simulink model "TubeFurnaceSim_2023b"  (R2023b)
settings: Solver=VariableStepAuto  StartTime=0.0  StopTime=240  FixedStep=0.001  RelTol=1e-3
values from neighbouring files (symbols this model uses):
  a_density = 1.225    [TubeFurnace.m]
  a_heat_cap = 1005    [TubeFurnace.m]
  ambient_temp = 25    [TubeFurnace.m]
  current = 15    [TubeFurnace.m]
  g = 9.81    [TubeFurnace.m]
  heat_eff = 0.85    [TubeFurnace.m]
  i_resist_cond = log((q_inner_dia/2 + i_thickness) / (q_inner_dia/2)) / (2*pi*i_therm_cond*q_length)    [TubeFurnace.m]
  k_d = 0    [TubeFurnace.m]
  k_i = 0    [TubeFurnace.m]
  k_p = 0.5    [TubeFurnace.m]
  q_emis = 0.8    [TubeFurnace.m]
  q_inner_dia = 20    [TubeFurnace.m]
  q_inner_sa = q_length * pi * (q_inner_dia / 2000)    (= 0.00957557440814)    [TubeFurnace.m]
  q_length = 1 * ft_to_m    (= 0.3048)    [TubeFurnace.m]
  stefan = 5.67*10^-8    (= 5.67e-08)    [TubeFurnace.m]
  w_tot_resist = w_resist * w_length / 100    (= 6.56167979003)    [TubeFurnace.m]
libraries: slpidlib x1
settings Model: Creator=Jason Kwok  LastModifiedBy=jason
settings RTWCC: GPUComputeCapability=5.0

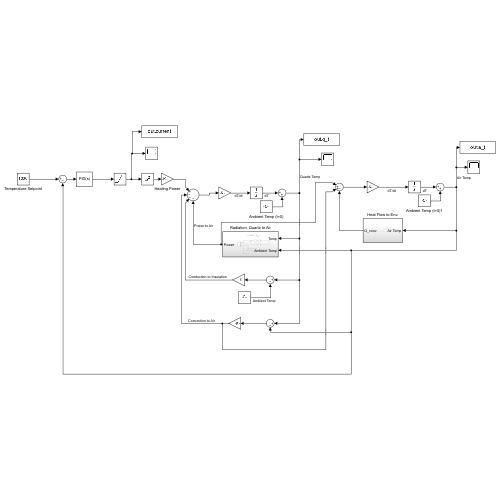
[thumbnail: Simulink's stored preview of the top-level diagram]
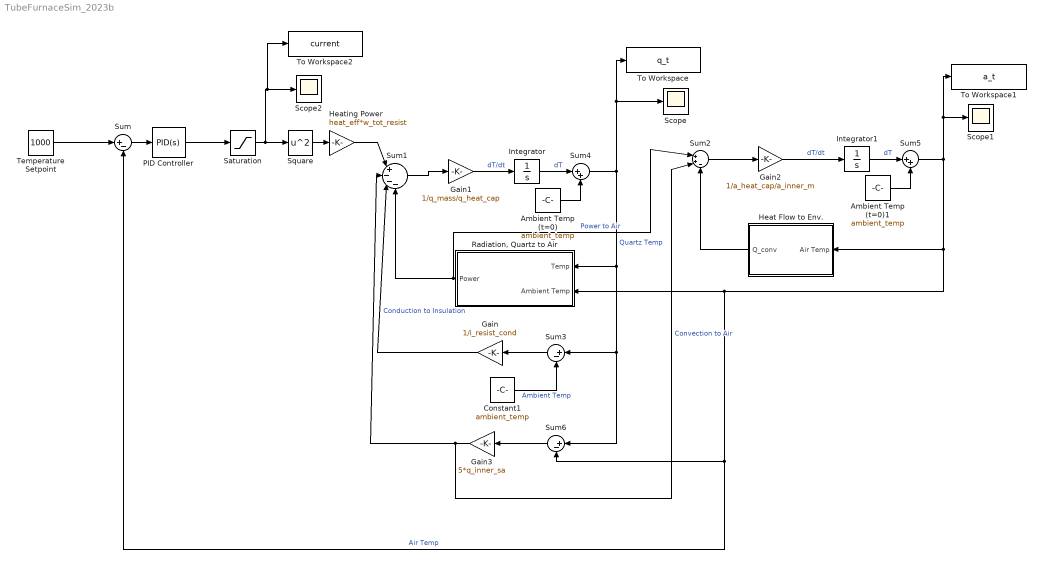
== system TubeFurnaceSim_2023b ==
  Ambient Temp (t=0) : Constant  Value=ambient_temp
  Ambient Temp (t=0)1 : Constant  Value=ambient_temp
  Constant1 : Constant  Value=ambient_temp
  Gain : Gain  Gain=1/i_resist_cond
  Gain1 : Gain  Gain=1/q_mass/q_heat_cap
  Gain2 : Gain  Gain=1/a_heat_cap/a_inner_m
  Gain3 : Gain  Gain=5*q_inner_sa
  Heat Flow to Env. : Subsystem
  Heating Power : Gain  Gain=heat_eff*w_tot_resist
  Integrator : Integrator
  Integrator1 : Integrator
  PID Controller : slpidlib/PID Controller  Controller=PID  Form=Parallel  TimeDomain=Continuous-time  UseExternalTs=off  SampleTime=-1  IntegratorMethod=Forward Euler  FilterMethod=Forward Euler  ControllerParametersSource=internal  P=k_p  I=k_i  UseKiTs=off  D=k_d  N=100  UseFilter=on  TunerSelectOption=Transfer Function Based (PID Tuner App)  InitialConditionSource=internal  InitialConditionForIntegrator=0  InitialConditionForFilter=0  DifferentiatorICPrevScaledInput=0  ExternalReset=none  TrackingMode=off  Kt=1  LimitOutput=off  SatLimitsSource=internal  UpperSaturationLimit=inf  LowerSaturationLimit=-inf  LinearizeAsGain=on  AntiWindupMode=none  Kb=1  LimitIntegrator=off  UpperIntegratorSaturationLimit=inf  LowerIntegratorSaturationLimit=-inf  POutMin=[]  POutMax=[]  IOutMin=[]  IOutMax=[]  DOutMin=[]  DOutMax=[]  NOutMin=[]  NOutMax=[]  SumOutMin=[]  SumOutMax=[]  SaturationOutMin=[]  SaturationOutMax=[]  PParamMin=[]  PParamMax=[]  IParamMin=[]  IParamMax=[]  DParamMin=[]  DParamMax=[]  NParamMin=[]  NParamMax=[]  KbParamMin=[]  KbParamMax=[]  KtParamMin=[]  KtParamMax=[]  KbOutMin=[]  KbOutMax=[]  KtOutMin=[]  KtOutMax=[]  IntegratorOutMin=[]  IntegratorOutMax=[]  FilterOutMin=[]  FilterOutMax=[]  SumI1OutMin=[]  SumI1OutMax=[]  SumI2OutMin=[]  SumI2OutMax=[]  SumI3OutMin=[]  SumI3OutMax=[]  SumI4OutMin=[]  SumI4OutMax=[]  SumDOutMin=[]  SumDOutMax=[]  DifferentiatorOutMin=[]  DifferentiatorOutMax=[]  FilterDiffOutCoefMin=[]  FilterDiffOutCoefMax=[]  ReciprocalOutMin=[]  ReciprocalOutMax=[]  SumDenOutMin=[]  SumDenOutMax=[]  SumNumOutMin=[]  SumNumOutMax=[]  DivideOutMin=[]  DivideOutMax=[]  UdiffTsProdOutMin=[]  UdiffTsProdOutMax=[]  NTsProdOutMin=[]  NTsProdOutMax=[]  UintegralTsProdOutMin=[]  UintegralTsProdOutMax=[]  UngainTsProdOutMin=[]  UngainTsProdOutMax=[]  ClampingZeroOutDataTypeStr=Inherit: Inherit via back propagation  ClampingZeroOutMin=[]  ClampingZeroOutMax=[]  FilterDenConstantOutDataTypeStr=Inherit: Inherit via back propagation  FilterDenConstantOutMin=[]  FilterDenConstantOutMax=[]  PCopyOutDataTypeStr=Inherit: Inherit via back propagation  PCopyOutMin=[]  PCopyOutMax=[]  NCopyOutDataTypeStr=Inherit: Inherit via back propagation  NCopyOutMin=[]  NCopyOutMax=[]  IntegratorContinuousStateAttributes=''  IntegratorStateMustResolveToSignalObject=off  IntegratorRTWStateStorageClass=Auto  FilterContinuousStateAttributes=''  FilterStateMustResolveToSignalObject=off  FilterRTWStateStorageClass=Auto  ParallelPVariant=InternalParameters  IdealPVariant=Disabled  IVariant=InternalParameters  DVariant=InternalParameters  IntegratorVariant=Continuous  SatVariant=Disabled  AWVariant=Passthrough  PCopyVariant=Disabled  TRVariant=Disabled  FdbkBlocksVariant=Forward  IdealPFdbkVariant=Disabled  SatFdbkVariant=Disabled  DerivativeFilterVariant=ContFilter  NVariant=InternalParameters  NCopyVariant=Disabled  FilterICVariant=InternalICsFilter  IntegratorICVariant=InternalICs  ExternalResetVariant=Disabled  TRSumVariant=Passthrough  SumFdbkVariant=Disabled  SumVariant=Sum_PID  TsampFilterVariant=InternalTs  TsampNgainVariant=Passthrough  TsampIntegralVariant=Disabled_SignalSpec  ExternalSaturationOutDataTypeStr=Inherit: Same as second input
  "Radiation, Quartz to Air" : Subsystem
  Saturation : Saturate  UpperLimit=current  LowerLimit=0
  Scope : Scope
  Scope1 : Scope
  Scope2 : Scope
  Square : Math  Operator=square
  Sum : Sum  Inputs=|+-
  Sum1 : Sum  Inputs=|+---
  Sum2 : Sum  Inputs=|++-
  Sum3 : Sum  Inputs=|+-
  Sum4 : Sum  Inputs=|++
  Sum5 : Sum  Inputs=|++
  Sum6 : Sum  Inputs=|+-
  Temperature Setpoint : Constant  Value=1000
  To Workspace : ToWorkspace  VariableName=q_t  SaveFormat=Timeseries  SampleTime=-1
  To Workspace1 : ToWorkspace  VariableName=a_t  SaveFormat=Timeseries  SampleTime=-1
  To Workspace2 : ToWorkspace  VariableName=current  SaveFormat=Timeseries  SampleTime=-1
  wires:
  Temperature Setpoint/1 -> Sum/1
  Sum/1 -> PID Controller/1
  Sum1/1 -> Gain1/1
  Heating Power/1 -> Sum1/1
  Integrator/1 -> Sum4/1  "dT"
  "Radiation, Quartz to Air"/1(Power) -> Sum1/4, Sum2/1  "Power to Air"
  Gain1/1 -> Integrator/1  "dT/dt"
  Sum2/1 -> Gain2/1
  Gain2/1 -> Integrator1/1  "dT/dt"
  Gain/1 -> Sum1/3  "Conduction to Insulation"
  Sum3/1 -> Gain/1
  Constant1/1 -> Sum3/2  "Ambient Temp"
  Saturation/1 -> Square/1, To Workspace2/1, Scope2/1
  Heat Flow to Env./1(Q_conv) -> Sum2/3
  Sum4/1 -> Sum6/1, Sum3/1, "Radiation, Quartz to Air"/1(Temp), Scope/1, To Workspace/1  "Quartz Temp"
  Ambient Temp (t=0)/1 -> Sum4/2
  Integrator1/1 -> Sum5/1  "dT"
  Ambient Temp (t=0)1/1 -> Sum5/2
  Sum5/1 -> To Workspace1/1, Scope1/1, "Radiation, Quartz to Air"/2(Ambient Temp), Sum6/2, Sum/2, Heat Flow to Env./1(Air Temp)  "Air Temp"
  Gain3/1 -> Sum2/2, Sum1/2  "Convection to Air"
  Sum6/1 -> Gain3/1
  Square/1 -> Heating Power/1
  PID Controller/1 -> Saturation/1

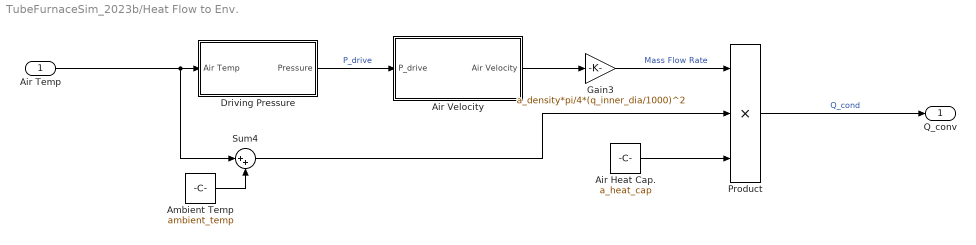
== system TubeFurnaceSim_2023b/Heat Flow to Env. ==
  Air Temp : Inport
  Air Heat Cap. : Constant  Value=a_heat_cap
  Air Velocity : Subsystem
  Ambient Temp : Constant  Value=ambient_temp
  Driving Pressure : Subsystem
  Gain3 : Gain  Gain=a_density*pi/4*(q_inner_dia/1000)^2
  Product : Product  Inputs=3
  Sum4 : Sum  Inputs=|++
  Q_conv : Outport
  wires:
  Air Temp/1 -> Sum4/1, Driving Pressure/1(Air Temp)
  Product/1 -> Q_conv/1  "Q_cond"
  Sum4/1 -> Product/2
  Driving Pressure/1(Pressure) -> Air Velocity/1(P_drive)  "P_drive"
  Ambient Temp/1 -> Sum4/2
  Gain3/1 -> Product/1  "Mass Flow Rate"
  Air Velocity/1(Air Velocity) -> Gain3/1
  Air Heat Cap./1 -> Product/3

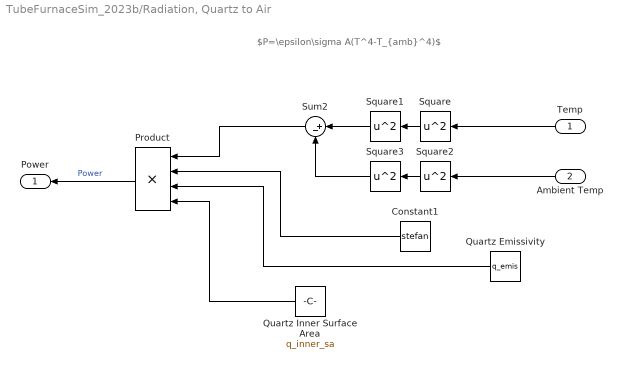
== system TubeFurnaceSim_2023b/Radiation, Quartz to Air ==
  note: $P=\epsilon\sigma A(T^4-T_{amb}^4)$
  Temp : Inport
  Ambient Temp : Inport  Port=2
  Constant1 : Constant  Value=stefan
  Product : Product  Inputs=4
  Quartz Emissivity : Constant  Value=q_emis
  Quartz Inner Surface Area : Constant  Value=q_inner_sa
  Square{,1..3} (4 alike) : Math  Operator=square
  Sum2 : Sum  Inputs=|+-
  Power : Outport
  wires:
  Ambient Temp/1 -> Square2/1
  Square1/1 -> Sum2/1
  Square2/1 -> Square3/1
  Square/1 -> Square1/1
  Sum2/1 -> Product/1
  Product/1 -> Power/1  "Power"
  Constant1/1 -> Product/2
  Quartz Emissivity/1 -> Product/3
  Square3/1 -> Sum2/2
  Temp/1 -> Square/1
  Quartz Inner Surface Area/1 -> Product/4

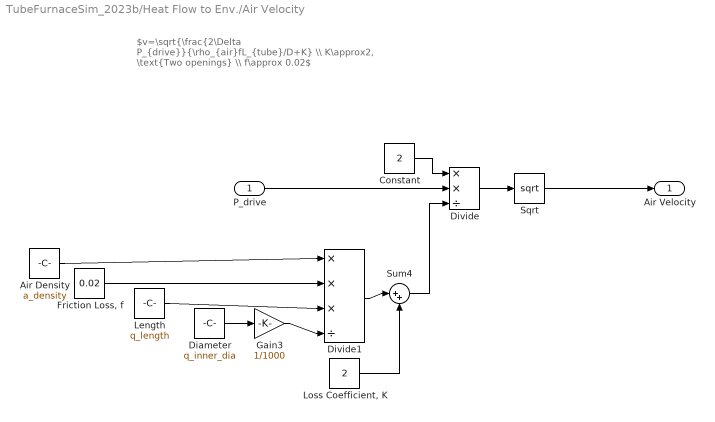
== system TubeFurnaceSim_2023b/Heat Flow to Env./Air Velocity ==
  note: $v=\sqrt{\frac{2\Delta P_{drive}}{\rho_{air}fL_{tube}/D+K} \\ K\approx2, \text{Two openings} \\ f\approx 0.02$
  P_drive : Inport
  Air Density : Constant  Value=a_density
  Constant : Constant  Value=2
  Diameter : Constant  Value=q_inner_dia
  Divide : Product  Inputs=**/
  Divide1 : Product  Inputs=***/
  "Friction Loss, f" : Constant  Value=0.02
  Gain3 : Gain  Gain=1/1000
  Length : Constant  Value=q_length
  "Loss Coefficient, K" : Constant  Value=2
  Sqrt : Sqrt
  Sum4 : Sum  Inputs=|++
  Air Velocity : Outport
  wires:
  Air Density/1 -> Divide1/1
  Sum4/1 -> Divide/3
  "Friction Loss, f"/1 -> Divide1/2
  Length/1 -> Divide1/3
  Divide1/1 -> Sum4/1
  Diameter/1 -> Gain3/1
  Constant/1 -> Divide/1
  Divide/1 -> Sqrt/1
  Gain3/1 -> Divide1/4
  "Loss Coefficient, K"/1 -> Sum4/2
  Sqrt/1 -> Air Velocity/1
  P_drive/1 -> Divide/2

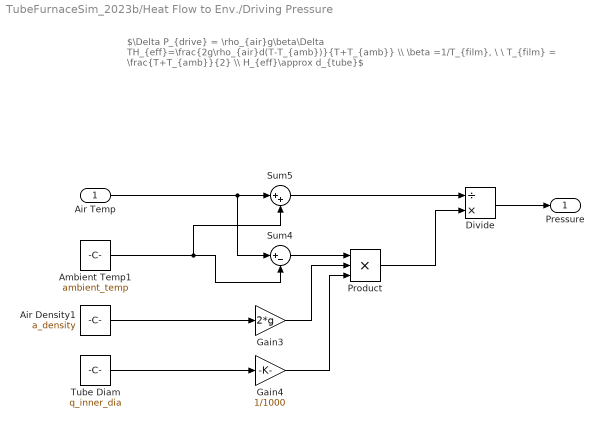
== system TubeFurnaceSim_2023b/Heat Flow to Env./Driving Pressure ==
  note: $\Delta P_{drive} = \rho_{air}g\beta\Delta TH_{eff}=\frac{2g\rho_{air}d(T-T_{amb})}{T+T_{amb}} \\ \beta =1/T_{film}, \ \ T_{film} = \frac{T+T_{amb}}{2} \\ H_{eff}\approx d_{tube}$
  Air Temp : Inport
  Air Density1 : Constant  Value=a_density
  Ambient Temp1 : Constant  Value=ambient_temp
  Divide : Product  Inputs=/*
  Gain3 : Gain  Gain=2*g
  Gain4 : Gain  Gain=1/1000
  Product : Product  Inputs=3
  Sum4 : Sum  Inputs=|+-
  Sum5 : Sum  Inputs=|++
  Tube Diam : Constant  Value=q_inner_dia
  Pressure : Outport
  wires:
  Sum4/1 -> Product/1
  Gain4/1 -> Product/3
  Air Temp/1 -> Sum4/1, Sum5/1
  Tube Diam/1 -> Gain4/1
  Product/1 -> Divide/2
  Sum5/1 -> Divide/1
  Gain3/1 -> Product/2
  Ambient Temp1/1 -> Sum4/2, Sum5/2
  Divide/1 -> Pressure/1
  Air Density1/1 -> Gain3/1
